simulink model "yaw"  (R2024b)
settings: Solver=VariableStepAuto  StartTime=0.0  StopTime=10.0  RelTol=1e-3
settings Model: Creator=Zohaib  LastModifiedBy=Zohaib

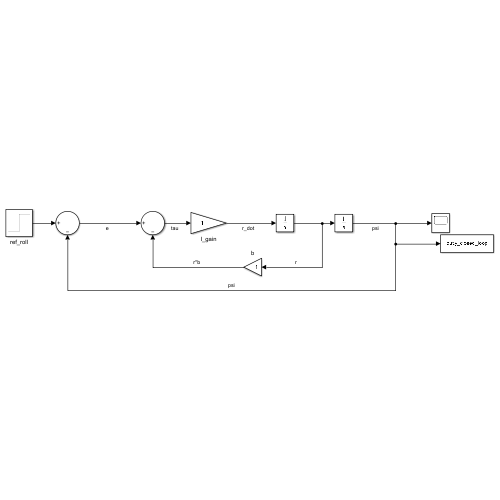
[thumbnail: Simulink's stored preview of the top-level diagram]
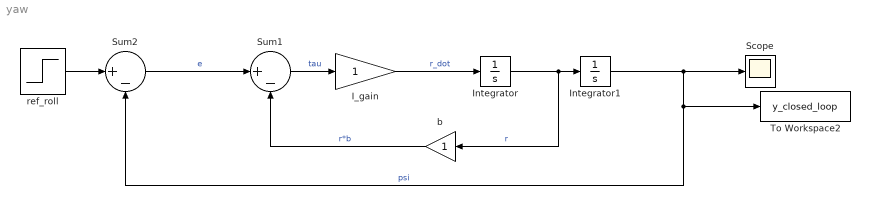
== system yaw ==
  I_gain : Gain
  Integrator : Integrator
  Integrator1 : Integrator
  Scope : Scope
  Sum1 : Sum  Inputs=|+-
  Sum2 : Sum  Inputs=|+-
  To Workspace2 : ToWorkspace  VariableName=y_closed_loop  SaveFormat=Timeseries  SampleTime=-1
  b : Gain
  ref_roll : Step  Time=0  SampleTime=0
  wires:
  Sum1/1 -> I_gain/1  "tau"
  Sum2/1 -> Sum1/1  "e"
  Integrator1/1 -> Sum2/2, To Workspace2/1, Scope/1  "psi"
  b/1 -> Sum1/2  "r*b"
  ref_roll/1 -> Sum2/1
  I_gain/1 -> Integrator/1  "r_dot"
  Integrator/1 -> b/1, Integrator1/1  "r"
